simulink model "fuel_cell_1cell"  (R2024a)
settings: Solver=VariableStepAuto  StartTime=0.0  StopTime=10  RelTol=1e-3
values from neighbouring files (symbols this model uses):
  A_fc_m2 = 25e-4    (= 0.0025)    [test.m]
  b11 = 0.5139    [test.m]
  b12 = 0.326    [test.m]
  B_0 = 2.9294976e-09    [test.m]
  c_0 = 1.012286e-07    [test.m]
  dG_data = [-237.2 -227.0 -225.2 -220.4 -210.3 -199.6 -188.6 -177.4]*1000    [test.m]
  F = 96485    [test.m]
  Imax = 0.25    [test.m]
  M_O2 = 32    [test.m]
  M_vapor = 18    [test.m]
  n_d = 1    [test.m]
  p_tank = 6    [test.m]
  T_data = [298 353 373 473 673 873 1073 1273]    [test.m]
  t_m_m = 178e-6    (= 0.000178)    [test.m]
  xi1_0 = -0.88417943    [test.m]
  xi2_0 = 0.010610204    [test.m]
  xi3_0 = 5.0249916e-04    (= 0.00050249916)    [test.m]
  xi4_0 = -1.261376e-03    (= -0.001261376)    [test.m]
libraries: simulink x2, slpidlib x1
settings Model: Creator=Lagha  LastModifiedBy=Lagha

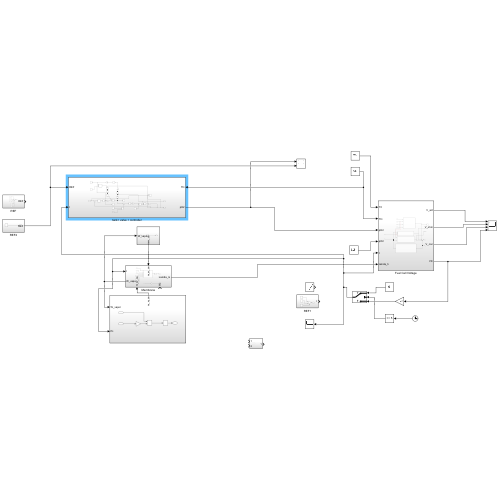
[thumbnail: Simulink's stored preview of the top-level diagram]
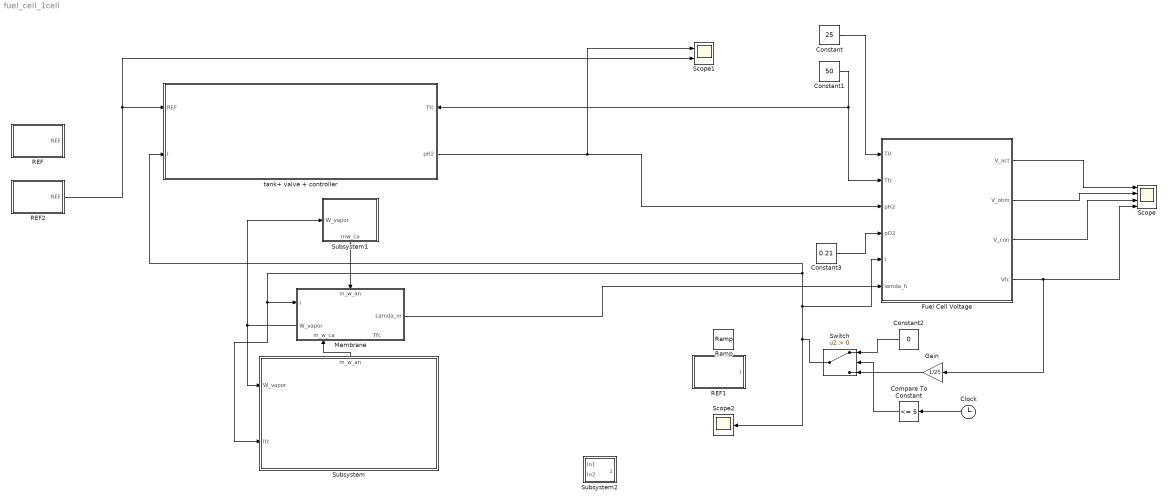
== system fuel_cell_1cell ==
  Clock : Clock
  Compare To Constant : simulink/Logic and Bit Operations/Compare To Constant  relop=<=  const=5  OutDataTypeStr=boolean
  Constant : Constant  Value=25
  Constant1 : Constant  Value=50
  Constant2 : Constant  Value=0
  Constant3 : Constant  Value=0.21
  Fuel Cell Voltage : Subsystem
  Gain : Gain  Gain=1/25
  Membrane : Subsystem
      settings: PortSchema="{\"entries\":[{\"content\":{\"sides\":[{\"content\":{\"connectorIds\":[\"In1\",\"Out2\"]},\"type\":\"ConnectorPlacement.EquallySpacedRectSide\",\"uuid\":\"d761c1e9-1ccf-4514-90a1-cbf676d5b141\"},{\"content\":{\"connectorIds\":[\"Out1\"],\"side\":\"RIGHT\"},\"type\":\"ConnectorPlacement.EquallySpacedRectSide\",\"uuid\":\"4ebf0d6c-6255-4c98-92ba-5e76677595a5\"},{\"content\":{\"connectorIds\":[\"In2\"],\"side\":\"TOP\"},\"type\":\"ConnectorPlacement.EquallySpacedRectSide\",\"uuid\":\"3294e2c8-05cd-412a-a5c6-a701570d0b74\"},{\"content\":{\"connectorIds\":[\"In3\",\"In4\"],\"side\":\"BOTTOM\"},\"type\":\"ConnectorPlacement.EquallySpacedRectSide\",\"uuid\":\"5eaf2422-cf7b-4bb8-bd76-8cd1db5b1f32\"}]},\"type\":\"ConnectorPlacement.EquallySpacedConnector\",\"uuid\":\"213a923d-75a6-4d49-be69-6e1a866eed78\"}],\"packageUris\":[\"http://schema.mathworks.com/mf0/Connector/R2020b\"],\"version\":\"1.0\"}"
  REF : Subsystem
  REF1 : Subsystem
  REF2 : Subsystem
  Ramp : simulink/Sources/Ramp  slope=0.25/15  start=0  InitialOutput=0
  Scope : Scope  NumInputPorts=4
  Scope1 : Scope  NumInputPorts=2
  Scope2 : Scope
  Subsystem : Subsystem
      settings: PortSchema="{\"entries\":[{\"content\":{\"sides\":[{\"content\":{\"connectorIds\":[\"In1\",\"In2\"]},\"type\":\"ConnectorPlacement.EquallySpacedRectSide\",\"uuid\":\"7cd8950e-2e27-4839-b109-cd3de7054c1e\"},{\"content\":{\"side\":\"RIGHT\"},\"type\":\"ConnectorPlacement.EquallySpacedRectSide\",\"uuid\":\"410f8dcc-6135-4046-8699-ffc709e8fed5\"},{\"content\":{\"connectorIds\":[\"Out1\"],\"side\":\"TOP\"},\"type\":\"ConnectorPlacement.EquallySpacedRectSide\",\"uuid\":\"dcdc622b-d54c-4c8e-b867-9e21d2b73c1e\"}]},\"type\":\"ConnectorPlacement.EquallySpacedConnector\",\"uuid\":\"28a1dbba-7a8d-44df-8950-32906d1b9d95\"}],\"packageUris\":[\"http://schema.mathworks.com/mf0/Connector/R2020b\"],\"version\":\"1.0\"}"
  Subsystem1 : Subsystem
      settings: PortSchema="{\"entries\":[{\"content\":{\"sides\":[{\"content\":{\"connectorIds\":[\"In1\"]},\"type\":\"ConnectorPlacement.EquallySpacedRectSide\",\"uuid\":\"d761c1e9-1ccf-4514-90a1-cbf676d5b141\"},{\"content\":{\"side\":\"RIGHT\"},\"type\":\"ConnectorPlacement.EquallySpacedRectSide\",\"uuid\":\"4ebf0d6c-6255-4c98-92ba-5e76677595a5\"},{\"content\":{\"side\":\"TOP\"},\"type\":\"ConnectorPlacement.EquallySpacedRectSide\",\"uuid\":\"3294e2c8-05cd-412a-a5c6-a701570d0b74\"},{\"content\":{\"connectorIds\":[\"Out1\"],\"side\":\"BOTTOM\"},\"type\":\"ConnectorPlacement.EquallySpacedRectSide\",\"uuid\":\"a1a8a6cf-412b-42b1-bf45-b39bb9e9fb91\"}]},\"type\":\"ConnectorPlacement.EquallySpacedConnector\",\"uuid\":\"213a923d-75a6-4d49-be69-6e1a866eed78\"}],\"packageUris\":[\"http://schema.mathworks.com/mf0/Connector/R2020b\"],\"version\":\"1.0\"}"
  Subsystem2 : Subsystem
  Switch : Switch  Criteria=u2 > Threshold  SaturateOnIntegerOverflow=off  InputSameDT=off
  tank+ valve + controller : Subsystem
      settings: PortSchema="{\"entries\":[{\"content\":{\"sides\":[{\"content\":{\"connectorIds\":[\"In1\",\"In2\"]},\"type\":\"ConnectorPlacement.EquallySpacedRectSide\",\"uuid\":\"3ef60475-1bce-4d1a-9494-b62c0b89f9b8\"},{\"content\":{\"connectorIds\":[\"In3\",\"Out1\"],\"side\":\"RIGHT\"},\"type\":\"ConnectorPlacement.EquallySpacedRectSide\",\"uuid\":\"35db6bc9-751f-4d20-af99-50f6673c6172\"},{\"content\":{\"side\":\"TOP\"},\"type\":\"ConnectorPlacement.EquallySpacedRectSide\",\"uuid\":\"904b1159-5fc4-4a2c-b5dc-6990e1e9e7c6\"},{\"content\":{\"side\":\"BOTTOM\"},\"type\":\"ConnectorPlacement.EquallySpacedRectSide\",\"uuid\":\"2d5692df-ffba-4243-9114-bb194a646cc0\"}]},\"type\":\"ConnectorPlacement.EquallySpacedConnector\",\"uuid\":\"0a2ad4d5-4029-4127-bc12-9c854306c0dc\"}],\"packageUris\":[\"http://schema.mathworks.com/mf0/Connector/R2020b\"],\"version\":\"1.0\"}"
  wires:
  Constant/1 -> Fuel Cell Voltage/1(T0)
  Constant3/1 -> Fuel Cell Voltage/4(pO2)
  Fuel Cell Voltage/1(V_act) -> Scope/1
  Fuel Cell Voltage/2(V_ohm) -> Scope/2
  Fuel Cell Voltage/3(V_con) -> Scope/3
  Fuel Cell Voltage/4(Vfc) -> Gain/1, Scope/4
  Clock/1 -> Compare To Constant/1
  Compare To Constant/1 -> Switch/2
  Gain/1 -> Switch/3
  Constant2/1 -> Switch/1
  REF2/1(REF) -> Scope1/2, tank+ valve + controller/1(REF)
  Membrane/2(W_vapor) -> Subsystem/1(W_vapor), Subsystem1/1(W_vapor)
  Subsystem1/1(mw_ca) -> Membrane/2(m_w_an)
  Subsystem/1(m_w_an) -> Membrane/3(m_w_ca)
  Switch/1 -> tank+ valve + controller/2(I), Subsystem/2(Ifc), Membrane/1(I), Fuel Cell Voltage/5(I), Scope2/1
  Membrane/1(Lamda_m) -> Fuel Cell Voltage/6(lamda_h)
  Constant1/1 -> Fuel Cell Voltage/2(Tfc), tank+ valve + controller/3(Tfc)
  tank+ valve + controller/1(pH2) -> Scope1/1, Fuel Cell Voltage/3(pH2)

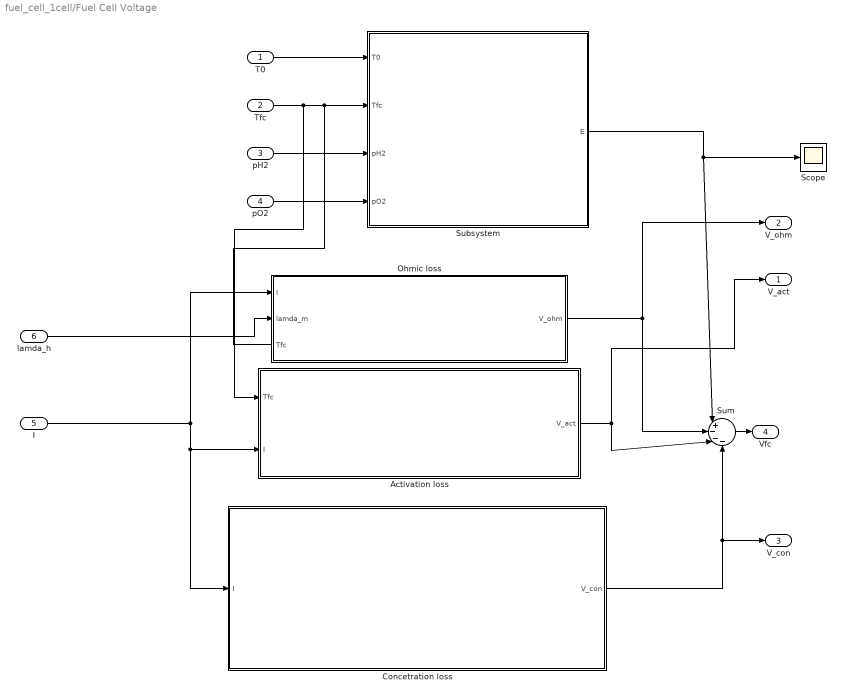
== system fuel_cell_1cell/Fuel Cell Voltage ==
  T0 : Inport
  Tfc : Inport  Port=2
  pH2 : Inport  Port=3
  pO2 : Inport  Port=4
  I : Inport  Port=5
  lamda_h : Inport  Port=6
  Activation loss : Subsystem
  Concetration loss : Subsystem
  Ohmic loss : Subsystem
  Scope : Scope
  Subsystem : Subsystem
  Sum : Sum  Inputs=|+---
  V_act : Outport
  V_ohm : Outport  Port=2
  V_con : Outport  Port=3
  Vfc : Outport  Port=4
  wires:
  Ohmic loss/1(V_ohm) -> V_ohm/1, Sum/2
  Activation loss/1(V_act) -> Sum/3, V_act/1
  Concetration loss/1(V_con) -> Sum/4, V_con/1
  Subsystem/1(E) -> Scope/1, Sum/1
  Sum/1 -> Vfc/1
  I/1 -> Concetration loss/1(I), Activation loss/2(I), Ohmic loss/1(I)
  T0/1 -> Subsystem/1(T0)
  Tfc/1 -> Activation loss/1(Tfc), Subsystem/2(Tfc)
  pH2/1 -> Subsystem/3(pH2)
  pO2/1 -> Subsystem/4(pO2)
  lamda_h/1 -> Ohmic loss/2(lamda_m)

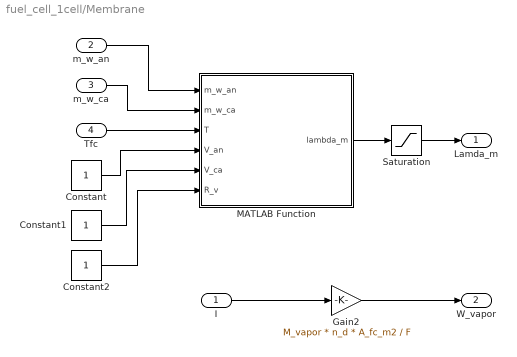
== system fuel_cell_1cell/Membrane ==
  I : Inport
  m_w_an : Inport  Port=2
  m_w_ca : Inport  Port=3
  Tfc : Inport  Port=4
  Constant : Constant
  Constant1 : Constant
  Constant2 : Constant
  Gain2 : Gain  Gain=M_vapor * n_d * A_fc_m2 / F
  MATLAB Function : MATLAB Function  TreatAsAtomicUnit=on
  Saturation : Saturate  UpperLimit=14  LowerLimit=1
  Lamda_m : Outport
  W_vapor : Outport  Port=2
  wires:
  Gain2/1 -> W_vapor/1
  I/1 -> Gain2/1
  Saturation/1 -> Lamda_m/1
  m_w_an/1 -> MATLAB Function/1(m_w_an)
  m_w_ca/1 -> MATLAB Function/2(m_w_ca)
  Tfc/1 -> MATLAB Function/3(T)
  Constant/1 -> MATLAB Function/4(V_an)
  Constant1/1 -> MATLAB Function/5(V_ca)
  Constant2/1 -> MATLAB Function/6(R_v)
  MATLAB Function/1(lambda_m) -> Saturation/1

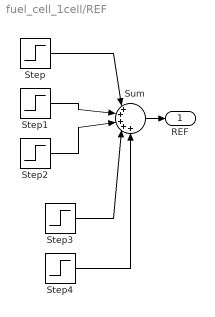
== system fuel_cell_1cell/REF ==
  Step : Step  Time=2  After=2  SampleTime=0
  Step1 : Step  Time=5  After=-0.5  SampleTime=0
  Step2 : Step  Time=7  After=0.3  SampleTime=0
  Step3 : Step  Time=9  After=-1  SampleTime=0
  Step4 : Step  Time=12  After=-0.7  SampleTime=0
  Sum : Sum  Inputs=|+++++
  REF : Outport
  wires:
  Step1/1 -> Sum/2
  Step/1 -> Sum/1
  Step2/1 -> Sum/3
  Sum/1 -> REF/1
  Step3/1 -> Sum/4
  Step4/1 -> Sum/5

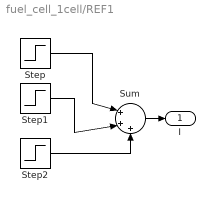
== system fuel_cell_1cell/REF1 ==
  Step : Step  Time=2  After=0.8/25  SampleTime=0
  Step1 : Step  Time=4  After=3  SampleTime=0
  Step2 : Step  Time=7  After=-6  SampleTime=0
  Sum : Sum  Inputs=|+++
  I : Outport
  wires:
  Step1/1 -> Sum/2
  Step/1 -> Sum/1
  Step2/1 -> Sum/3
  Sum/1 -> I/1

== system fuel_cell_1cell/REF2 ==
  Step : Step  After=2  SampleTime=0
  REF : Outport
  wires:
  Step/1 -> REF/1

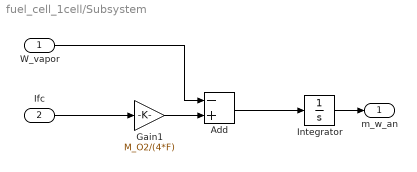
== system fuel_cell_1cell/Subsystem ==
  W_vapor : Inport
  Ifc : Inport  Port=2
  Add : Sum  Inputs=-+
  Gain1 : Gain  Gain=M_O2/(4*F)
  Integrator : Integrator
  m_w_an : Outport
  wires:
  Add/1 -> Integrator/1
  Gain1/1 -> Add/2
  W_vapor/1 -> Add/1
  Integrator/1 -> m_w_an/1
  Ifc/1 -> Gain1/1

== system fuel_cell_1cell/Subsystem1 ==
  W_vapor : Inport
  Integrator : Integrator
  mw_ca : Outport
  wires:
  W_vapor/1 -> Integrator/1
  Integrator/1 -> mw_ca/1

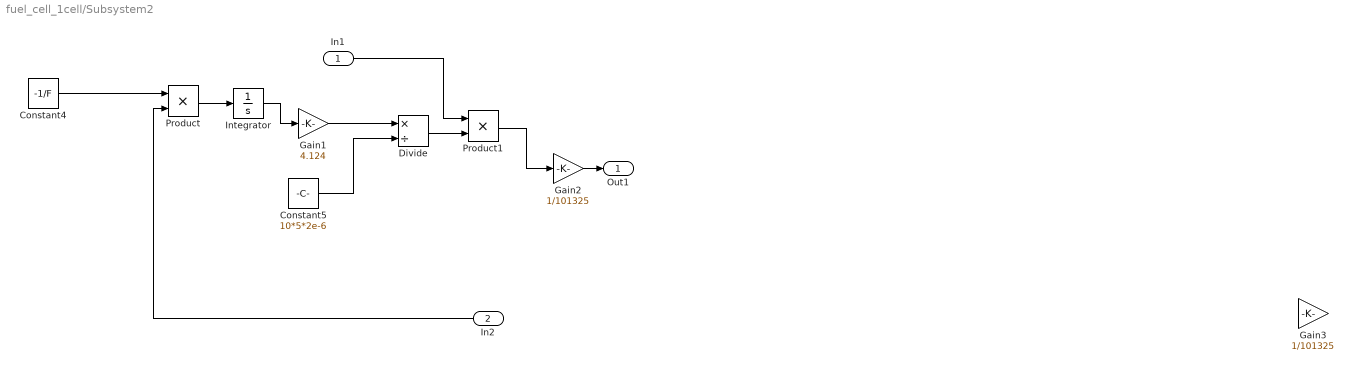
== system fuel_cell_1cell/Subsystem2 ==
  In1 : Inport
  In2 : Inport  Port=2
  Constant4 : Constant  Value=-1/F
  Constant5 : Constant  Value=10*5*2e-6
  Divide : Product  Inputs=*/
  Gain1 : Gain  Gain=4.124
  Gain2 : Gain  Gain=1/101325
  Gain3 : Gain  Gain=1/101325
  Integrator : Integrator  InitialCondition=0.1
  Product : Product
  Product1 : Product
  Out1 : Outport
  wires:
  Gain1/1 -> Divide/1
  Constant5/1 -> Divide/2
  In1/1 -> Product1/1
  Integrator/1 -> Gain1/1
  Divide/1 -> Product1/2
  In2/1 -> Product/2
  Product/1 -> Integrator/1
  Constant4/1 -> Product/1
  Gain2/1 -> Out1/1
  Product1/1 -> Gain2/1

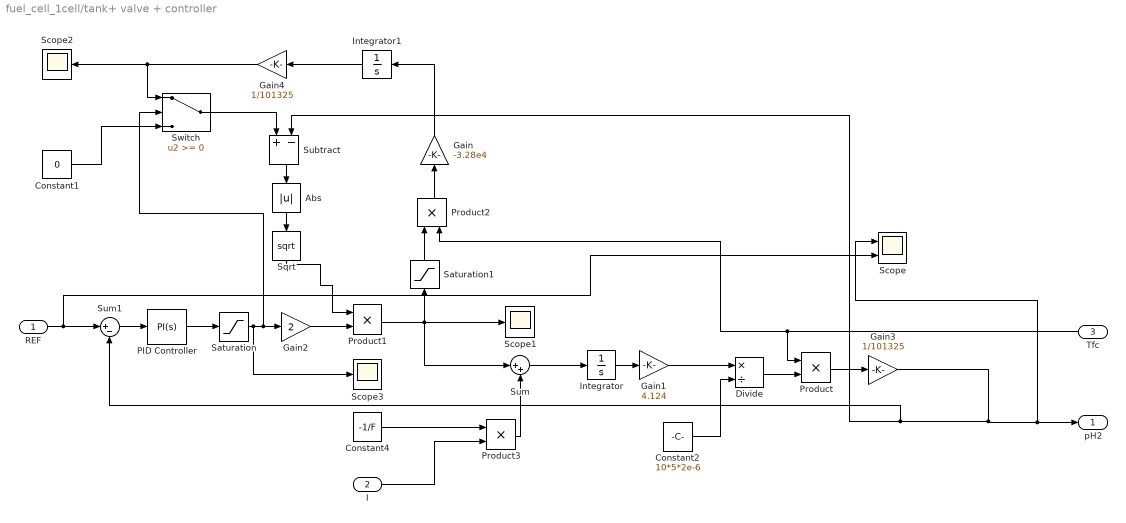
== system fuel_cell_1cell/tank+ valve + controller ==
  REF : Inport
  I : Inport  Port=2
  Tfc : Inport  Port=3
  Abs : Abs  SaturateOnIntegerOverflow=off
  Constant1 : Constant  Value=0
  Constant2 : Constant  Value=10*5*2e-6
  Constant4 : Constant  Value=-1/F
  Divide : Product  Inputs=*/
  Gain : Gain  Gain=-3.28e4
  Gain1 : Gain  Gain=4.124
  Gain2 : Gain  Gain=2
  Gain3 : Gain  Gain=1/101325
  Gain4 : Gain  Gain=1/101325
  Integrator : Integrator
  Integrator1 : Integrator  InitialCondition=p_tank*101325
  PID Controller : slpidlib/PID Controller  Controller=PI  Form=Parallel  TimeDomain=Continuous-time  UseExternalTs=off  SampleTime=-1  IntegratorMethod=Forward Euler  FilterMethod=Forward Euler  ControllerParametersSource=internal  P=0.0604304496668098  I=0.00637291626088388  UseKiTs=off  D=0  UseExternalDerivativeSource=off  N=100  UseFilter=on  TunerSelectOption=Transfer Function Based (PID Tuner App)  InitialConditionSource=internal  InitialConditionForIntegrator=0  InitialConditionForFilter=0  DifferentiatorICPrevScaledInput=0  ExternalReset=none  TrackingMode=off  Kt=1  LimitOutput=off  SatLimitsSource=internal  UpperSaturationLimit=inf  LowerSaturationLimit=-inf  LinearizeAsGain=on  AntiWindupMode=none  Kb=1  LimitIntegrator=off  UpperIntegratorSaturationLimit=inf  LowerIntegratorSaturationLimit=-inf  POutMin=[]  POutMax=[]  IOutMin=[]  IOutMax=[]  DOutMin=[]  DOutMax=[]  NOutMin=[]  NOutMax=[]  SumOutMin=[]  SumOutMax=[]  SaturationOutMin=[]  SaturationOutMax=[]  PParamMin=[]  PParamMax=[]  IParamMin=[]  IParamMax=[]  DParamMin=[]  DParamMax=[]  NParamMin=[]  NParamMax=[]  KbParamMin=[]  KbParamMax=[]  KtParamMin=[]  KtParamMax=[]  KbOutMin=[]  KbOutMax=[]  KtOutMin=[]  KtOutMax=[]  IntegratorOutMin=[]  IntegratorOutMax=[]  FilterOutMin=[]  FilterOutMax=[]  SumI1OutMin=[]  SumI1OutMax=[]  SumI2OutMin=[]  SumI2OutMax=[]  SumI3OutMin=[]  SumI3OutMax=[]  SumI4OutMin=[]  SumI4OutMax=[]  SumDOutMin=[]  SumDOutMax=[]  DifferentiatorOutMin=[]  DifferentiatorOutMax=[]  FilterDiffOutCoefMin=[]  FilterDiffOutCoefMax=[]  ReciprocalOutMin=[]  ReciprocalOutMax=[]  SumDenOutMin=[]  SumDenOutMax=[]  SumNumOutMin=[]  SumNumOutMax=[]  DivideOutMin=[]  DivideOutMax=[]  UdiffTsProdOutMin=[]  UdiffTsProdOutMax=[]  NTsProdOutMin=[]  NTsProdOutMax=[]  UintegralTsProdOutMin=[]  UintegralTsProdOutMax=[]  UngainTsProdOutMin=[]  UngainTsProdOutMax=[]  ClampingZeroOutDataTypeStr=Inherit: Inherit via back propagation  ClampingZeroOutMin=[]  ClampingZeroOutMax=[]  FilterDenConstantOutDataTypeStr=Inherit: Inherit via back propagation  FilterDenConstantOutMin=[]  FilterDenConstantOutMax=[]  PCopyOutDataTypeStr=Inherit: Inherit via back propagation  PCopyOutMin=[]  PCopyOutMax=[]  NCopyOutDataTypeStr=Inherit: Inherit via back propagation  NCopyOutMin=[]  NCopyOutMax=[]  IntegratorContinuousStateAttributes=''  IntegratorStateMustResolveToSignalObject=off  IntegratorRTWStateStorageClass=Auto  FilterContinuousStateAttributes=''  FilterStateMustResolveToSignalObject=off  FilterRTWStateStorageClass=Auto  ParallelPVariant=InternalParameters  IdealPVariant=Disabled  IVariant=InternalParameters  DVariant=Disabled  IntegratorVariant=Continuous  SatVariant=Disabled  AWVariant=Passthrough  PCopyVariant=Disabled  TRVariant=Disabled  FdbkBlocksVariant=Forward  IdealPFdbkVariant=Disabled  SatFdbkVariant=Disabled  DerivativeFilterVariant=Disabled  NVariant=Disabled  NCopyVariant=Disabled_SignalSpec  FilterICVariant=Disabled  IntegratorICVariant=InternalICs  ExternalResetVariant=Disabled  TRSumVariant=Passthrough  SumFdbkVariant=Disabled  SumVariant=Sum_PI  TsampFilterVariant=InternalTs  TsampNgainVariant=Passthrough  TsampIntegralVariant=Disabled_SignalSpec  ExternalSaturationOutDataTypeStr=Inherit: Same as second input  DerivativeSourceVariant=Disabled
  Product{,1..3} (4 alike) : Product
  Saturation : Saturate  UpperLimit=1  LowerLimit=-1
  Saturation1 : Saturate  UpperLimit=inf  LowerLimit=0
  Scope : Scope  NumInputPorts=2
  Scope1 : Scope
  Scope2 : Scope
  Scope3 : Scope
  Sqrt : Sqrt
  Subtract : Sum  Inputs=+-
  Sum : Sum  Inputs=|++
  Sum1 : Sum  Inputs=|+-
  Switch : Switch  SaturateOnIntegerOverflow=off  InputSameDT=off
  pH2 : Outport
  wires:
  Saturation/1 -> Scope3/1, Switch/2, Gain2/1
  Constant2/1 -> Divide/2
  Tfc/1 -> Product2/2, Product/1
  Gain2/1 -> Product1/2
  Sqrt/1 -> Product1/1
  Gain1/1 -> Divide/1
  Divide/1 -> Product/2
  Integrator/1 -> Gain1/1
  Product1/1 -> Sum/1, Scope1/1, Saturation1/1
  REF/1 -> Scope/2, Sum1/1
  Sum1/1 -> PID Controller/1
  Subtract/1 -> Abs/1
  Abs/1 -> Sqrt/1
  Product/1 -> Gain3/1
  Gain3/1 -> Sum1/2, Subtract/2, Scope/1, pH2/1
  PID Controller/1 -> Saturation/1
  Constant1/1 -> Switch/3
  Switch/1 -> Subtract/1
  Product2/1 -> Gain/1
  Gain/1 -> Integrator1/1
  Integrator1/1 -> Gain4/1
  Gain4/1 -> Scope2/1, Switch/1
  Saturation1/1 -> Product2/1
  Constant4/1 -> Product3/1
  Product3/1 -> Sum/2
  I/1 -> Product3/2
  Sum/1 -> Integrator/1

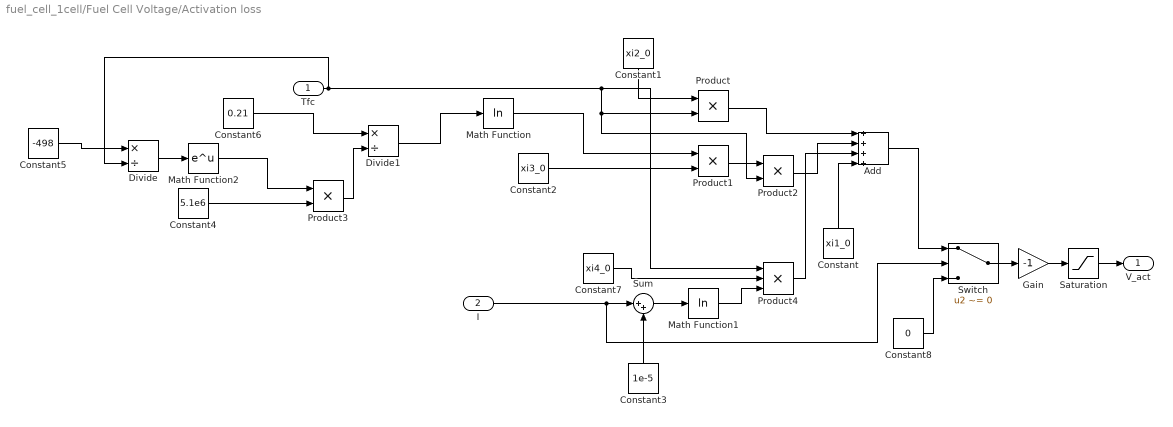
== system fuel_cell_1cell/Fuel Cell Voltage/Activation loss ==
  Tfc : Inport
  I : Inport  Port=2
  Add : Sum  Inputs=++++
  Constant : Constant  Value=xi1_0
  Constant1 : Constant  Value=xi2_0
  Constant2 : Constant  Value=xi3_0
  Constant3 : Constant  Value=1e-5
  Constant4 : Constant  Value=5.1e6
  Constant5 : Constant  Value=-498
  Constant6 : Constant  Value=0.21
  Constant7 : Constant  Value=xi4_0
  Constant8 : Constant  Value=0
  Divide : Product  Inputs=*/
  Divide1 : Product  Inputs=*/
  Gain : Gain  Gain=-1
  Math Function : Math  Operator=log
  Math Function1 : Math  Operator=log
  Math Function2 : Math
  Product{,1..3} (4 alike) : Product
  Product4 : Product  Inputs=3
  Saturation : Saturate  UpperLimit=inf  LowerLimit=0
  Sum : Sum  Inputs=|++
  Switch : Switch  Criteria=u2 ~= 0  SaturateOnIntegerOverflow=off  InputSameDT=off
  V_act : Outport
  wires:
  Tfc/1 -> Product4/1, Product2/2, Product/2, Divide/2
  Constant1/1 -> Product/1
  Product/1 -> Add/1
  Constant/1 -> Add/4
  Constant2/1 -> Product1/2
  Divide1/1 -> Math Function/1
  Math Function/1 -> Product1/1
  Product1/1 -> Product2/1
  Constant5/1 -> Divide/1
  Divide/1 -> Math Function2/1
  Math Function2/1 -> Product3/1
  Constant4/1 -> Product3/2
  Product3/1 -> Divide1/2
  Constant6/1 -> Divide1/1
  Product2/1 -> Add/2
  Math Function1/1 -> Product4/3
  Constant7/1 -> Product4/2
  Product4/1 -> Add/3
  I/1 -> Sum/1, Switch/2
  Switch/1 -> Gain/1
  Sum/1 -> Math Function1/1
  Constant3/1 -> Sum/2
  Add/1 -> Switch/1
  Constant8/1 -> Switch/3
  Gain/1 -> Saturation/1
  Saturation/1 -> V_act/1

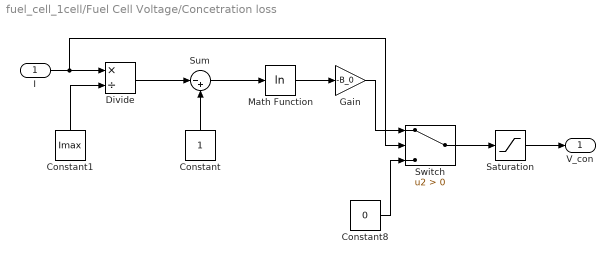
== system fuel_cell_1cell/Fuel Cell Voltage/Concetration loss ==
  I : Inport
  Constant : Constant
  Constant1 : Constant  Value=Imax
  Constant8 : Constant  Value=0
  Divide : Product  Inputs=*/
  Gain : Gain  Gain=-B_0
  Math Function : Math  Operator=log  OutputSignalType=real
  Saturation : Saturate  UpperLimit=inf  LowerLimit=0
  Sum : Sum  Inputs=|-+
  Switch : Switch  Criteria=u2 > Threshold  SaturateOnIntegerOverflow=off  InputSameDT=off
  V_con : Outport
  wires:
  Divide/1 -> Sum/1
  Sum/1 -> Math Function/1
  Math Function/1 -> Gain/1
  I/1 -> Switch/2, Divide/1
  Constant/1 -> Sum/2
  Constant1/1 -> Divide/2
  Constant8/1 -> Switch/3
  Gain/1 -> Switch/1
  Switch/1 -> Saturation/1
  Saturation/1 -> V_con/1

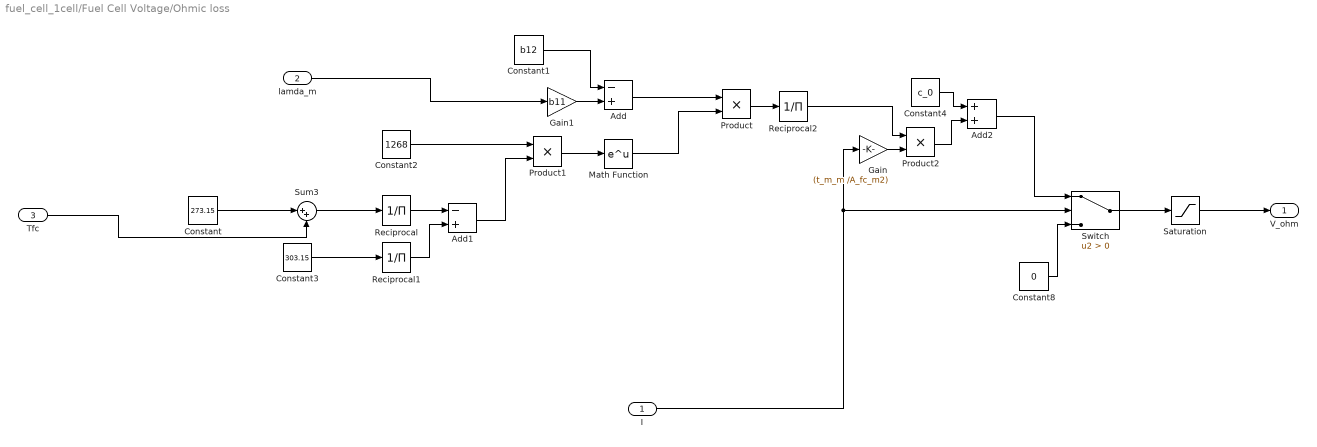
== system fuel_cell_1cell/Fuel Cell Voltage/Ohmic loss ==
  I : Inport
  lamda_m : Inport  Port=2
  Tfc : Inport  Port=3
  Add : Sum  Inputs=-+
  Add1 : Sum  Inputs=-+
  Add2 : Sum
  Constant : Constant  Value=273.15
  Constant1 : Constant  Value=b12
  Constant2 : Constant  Value=1268
  Constant3 : Constant  Value=303.15
  Constant4 : Constant  Value=c_0
  Constant8 : Constant  Value=0
  Gain : Gain  Gain=(t_m_m /A_fc_m2)
  Gain1 : Gain  Gain=b11
  Math Function : Math
  Product : Product
  Product1 : Product
  Product2 : Product
  Reciprocal : Product  Inputs=/
  Reciprocal1 : Product  Inputs=/
  Reciprocal2 : Product  Inputs=/
  Saturation : Saturate  UpperLimit=inf  LowerLimit=0
  Sum3 : Sum  Inputs=|++
  Switch : Switch  Criteria=u2 > Threshold  SaturateOnIntegerOverflow=off  InputSameDT=off
  V_ohm : Outport
  wires:
  I/1 -> Gain/1, Switch/2
  Constant8/1 -> Switch/3
  Switch/1 -> Saturation/1
  Saturation/1 -> V_ohm/1
  Add/1 -> Product/1
  Gain1/1 -> Add/2
  Constant1/1 -> Add/1
  lamda_m/1 -> Gain1/1
  Math Function/1 -> Product/2
  Constant3/1 -> Reciprocal1/1
  Reciprocal/1 -> Add1/1
  Reciprocal1/1 -> Add1/2
  Product1/1 -> Math Function/1
  Constant2/1 -> Product1/1
  Add1/1 -> Product1/2
  Product/1 -> Reciprocal2/1
  Gain/1 -> Product2/2
  Reciprocal2/1 -> Product2/1
  Constant4/1 -> Add2/1
  Product2/1 -> Add2/2
  Add2/1 -> Switch/1
  Constant/1 -> Sum3/1
  Tfc/1 -> Sum3/2
  Sum3/1 -> Reciprocal/1

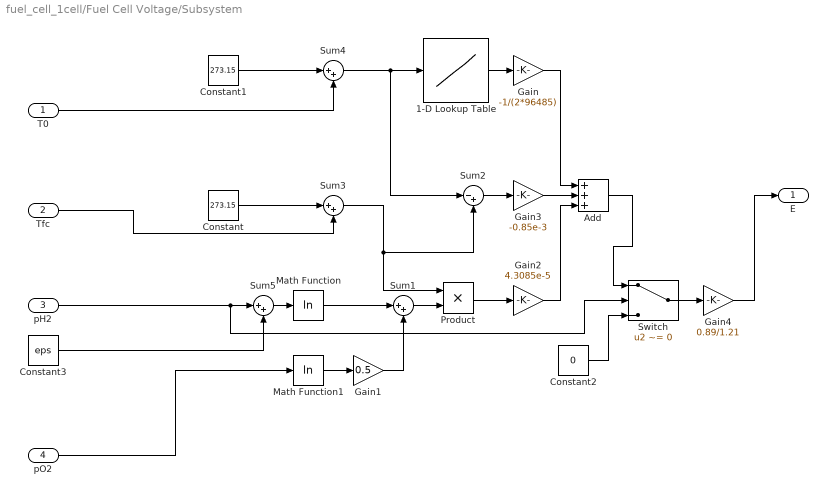
== system fuel_cell_1cell/Fuel Cell Voltage/Subsystem ==
  T0 : Inport
  Tfc : Inport  Port=2
  pH2 : Inport  Port=3
  pO2 : Inport  Port=4
  1-D Lookup Table : Lookup_n-D  NumberOfTableDimensions=1  BreakpointsForDimension1=T_data  Table=dG_data  ExtrapMethod=Clip  InternalRulePriority=Speed  RndMeth=Simplest
  Add : Sum  Inputs=+++
  Constant : Constant  Value=273.15
  Constant1 : Constant  Value=273.15
  Constant2 : Constant  Value=0
  Constant3 : Constant  Value=eps
  Gain : Gain  Gain=-1/(2*96485)
  Gain1 : Gain  Gain=0.5
  Gain2 : Gain  Gain=4.3085e-5
  Gain3 : Gain  Gain=-0.85e-3
  Gain4 : Gain  Gain=0.89/1.21
  Math Function : Math  Operator=log
  Math Function1 : Math  Operator=log
  Product : Product
  Sum{1,3..5} (4 alike) : Sum  Inputs=|++
  Sum2 : Sum  Inputs=|-+
  Switch : Switch  Criteria=u2 ~= 0  SaturateOnIntegerOverflow=off  InputSameDT=off
  E : Outport
  wires:
  T0/1 -> Sum4/2
  pO2/1 -> Math Function1/1
  Gain1/1 -> Sum1/2
  Sum3/1 -> Sum2/2, Product/1
  Sum1/1 -> Product/2
  1-D Lookup Table/1 -> Gain/1
  Gain/1 -> Add/1
  Sum2/1 -> Gain3/1
  Product/1 -> Gain2/1
  Gain2/1 -> Add/3
  Math Function1/1 -> Gain1/1
  Math Function/1 -> Sum1/1
  Gain3/1 -> Add/2
  Constant/1 -> Sum3/1
  Sum4/1 -> 1-D Lookup Table/1, Sum2/1
  Constant1/1 -> Sum4/1
  Tfc/1 -> Sum3/2
  pH2/1 -> Sum5/1, Switch/2
  Add/1 -> Switch/1
  Constant2/1 -> Switch/3
  Switch/1 -> Gain4/1
  Sum5/1 -> Math Function/1
  Constant3/1 -> Sum5/2
  Gain4/1 -> E/1

== matlab function fuel_cell_1cell/Membrane/MATLAB Function ==
  data: m_w_an input; lambda_m output; m_w_ca input; T input; V_an input; V_ca input; R_v input
function lambda_m = compute_lambda_m(m_w_an, m_w_ca, T, V_an, V_ca, R_v)

    % Saturation pressure [Pa] — Antoine approximation
    p_sat = 611.2 * exp(17.67 * (T - 273.15) / (T - 29.65));

    % Partial vapour pressures
    p_v_an = m_w_an * R_v * T / V_an;
    p_v_ca = m_w_ca * R_v * T / V_ca;

    % Relative humidities (clamped to [0, 1])
    phi_an = min(max(p_v_an / p_sat, 0), 1);
    phi_ca = min(max(p_v_ca / p_sat, 0), 1);

    % Springer sorption isotherm
    lambda_m = 0.5 * (springer(phi_an) + springer(phi_ca));
end

function lam = springer(a)
    a = min(max(a, 0), 1);
    lam = 0.043 + 17.81*a - 39.85*a^2 + 36.0*a^3;
end
